simulink model "bistaticAnalysisQuickReference"  (R2026a)
settings: Solver=VariableStepAuto
settings Model: Creator=pwilliam  LastModifiedBy=pwilliam

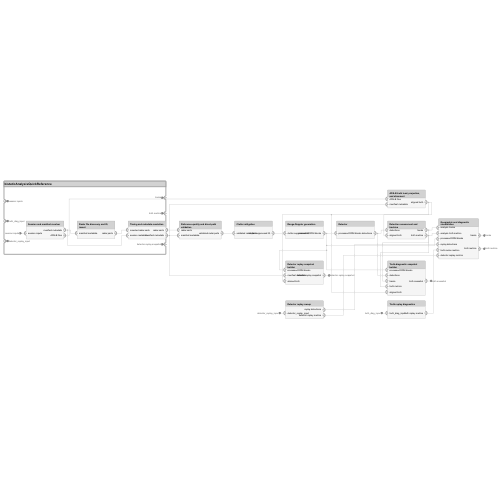
[thumbnail: Simulink's stored preview of the top-level diagram]
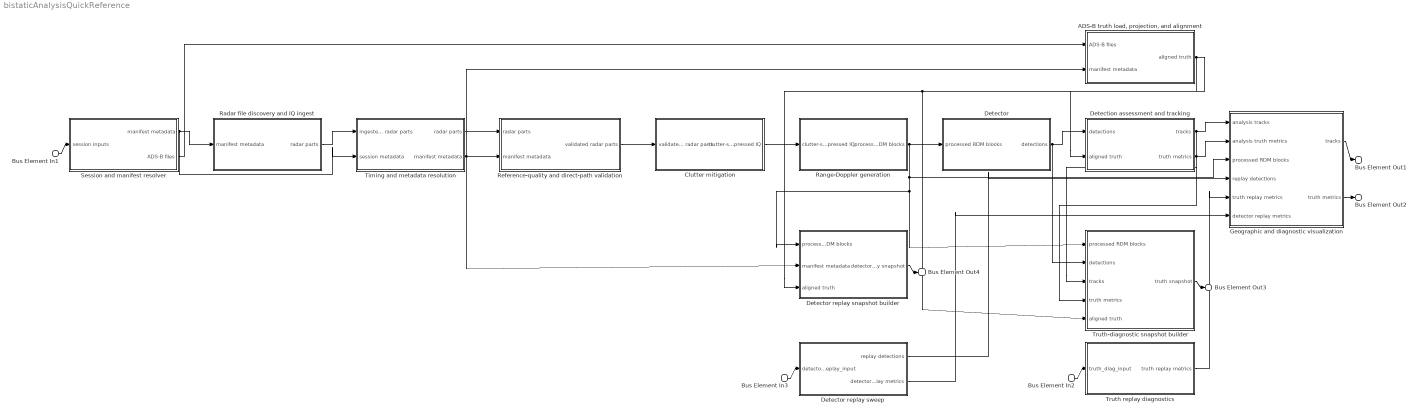
== system bistaticAnalysisQuickReference ==
  Bus Element In1 : Inport  PortName=session inputs
  Bus Element In2 : Inport  Port=2  PortName=truth_diag_input
  Bus Element In3 : Inport  Port=3  PortName=detector_replay_input
  "ADS-B truth load, projection, and alignment" : Subsystem
      settings: PortSchema="{\"entries\":[{\"content\":{\"headerSize\":26,\"margin\":15,\"minimumSpacing\":25,\"sides\":[{\"content\":{\"connectorIds\":[\"In1\",\"In2\"]},\"type\":\"ConnectorPlacement.EquallySpacedRectSide\",\"uuid\":\"3fc813c3-d4dd-4094-b53a-4fa94c312c6a\"},{\"content\":{\"connectorIds\":[\"Out1\"],\"side\":\"RIGHT\"},\"type\":\"ConnectorPlacement.EquallySpacedRectSide\",\"uuid\":\"6bc4ac0e-2abb-48a0-b5e3-8afa0902e8f2\"},{\"content\":{\"side\":\"TOP\"},\"type\":\"ConnectorPlacement.EquallySpacedRectSide\",\"uuid\":\"d3a5002a-6eae-4b58-9e29-e6d89f5a268f\"}]},\"type\":\"ConnectorPlacement.EquallySpacedConnector\",\"uuid\":\"d94812cc-5c4d-4681-a263-d12d583188a9\"}],\"packageUris\":[\"http://schema.mathworks.com/mf0/Connector/R2020b\"],\"version\":\"1.0\"}"
  Clutter mitigation : Subsystem
      settings: PortSchema="{\"entries\":[{\"content\":{\"headerSize\":26,\"margin\":15,\"minimumSpacing\":25,\"sides\":[{\"content\":{\"connectorIds\":[\"In1\"]},\"type\":\"ConnectorPlacement.EquallySpacedRectSide\",\"uuid\":\"3fc813c3-d4dd-4094-b53a-4fa94c312c6a\"},{\"content\":{\"connectorIds\":[\"Out1\"],\"side\":\"RIGHT\"},\"type\":\"ConnectorPlacement.EquallySpacedRectSide\",\"uuid\":\"6bc4ac0e-2abb-48a0-b5e3-8afa0902e8f2\"},{\"content\":{\"side\":\"TOP\"},\"type\":\"ConnectorPlacement.EquallySpacedRectSide\",\"uuid\":\"d3a5002a-6eae-4b58-9e29-e6d89f5a268f\"}]},\"type\":\"ConnectorPlacement.EquallySpacedConnector\",\"uuid\":\"d94812cc-5c4d-4681-a263-d12d583188a9\"}],\"packageUris\":[\"http://schema.mathworks.com/mf0/Connector/R2020b\"],\"version\":\"1.0\"}"
  Detection assessment and tracking : Subsystem
      settings: PortSchema="{\"entries\":[{\"content\":{\"headerSize\":26,\"margin\":15,\"minimumSpacing\":25,\"sides\":[{\"content\":{\"connectorIds\":[\"In1\",\"In2\"]},\"type\":\"ConnectorPlacement.EquallySpacedRectSide\",\"uuid\":\"3fc813c3-d4dd-4094-b53a-4fa94c312c6a\"},{\"content\":{\"connectorIds\":[\"Out1\",\"Out2\"],\"side\":\"RIGHT\"},\"type\":\"ConnectorPlacement.EquallySpacedRectSide\",\"uuid\":\"6bc4ac0e-2abb-48a0-b5e3-8afa0902e8f2\"},{\"content\":{\"side\":\"TOP\"},\"type\":\"ConnectorPlacement.EquallySpacedRectSide\",\"uuid\":\"d3a5002a-6eae-4b58-9e29-e6d89f5a268f\"}]},\"type\":\"ConnectorPlacement.EquallySpacedConnector\",\"uuid\":\"d94812cc-5c4d-4681-a263-d12d583188a9\"}],\"packageUris\":[\"http://schema.mathworks.com/mf0/Connector/R2020b\"],\"version\":\"1.0\"}"
  Detector : Subsystem
      settings: PortSchema="{\"entries\":[{\"content\":{\"headerSize\":26,\"margin\":15,\"minimumSpacing\":25,\"sides\":[{\"content\":{\"connectorIds\":[\"In1\"]},\"type\":\"ConnectorPlacement.EquallySpacedRectSide\",\"uuid\":\"3fc813c3-d4dd-4094-b53a-4fa94c312c6a\"},{\"content\":{\"connectorIds\":[\"Out1\"],\"side\":\"RIGHT\"},\"type\":\"ConnectorPlacement.EquallySpacedRectSide\",\"uuid\":\"6bc4ac0e-2abb-48a0-b5e3-8afa0902e8f2\"},{\"content\":{\"side\":\"TOP\"},\"type\":\"ConnectorPlacement.EquallySpacedRectSide\",\"uuid\":\"d3a5002a-6eae-4b58-9e29-e6d89f5a268f\"}]},\"type\":\"ConnectorPlacement.EquallySpacedConnector\",\"uuid\":\"d94812cc-5c4d-4681-a263-d12d583188a9\"}],\"packageUris\":[\"http://schema.mathworks.com/mf0/Connector/R2020b\"],\"version\":\"1.0\"}"
  Detector replay snapshot builder : Subsystem
      settings: PortSchema="{\"entries\":[{\"content\":{\"headerSize\":26,\"margin\":15,\"minimumSpacing\":25,\"sides\":[{\"content\":{\"connectorIds\":[\"In1\",\"In2\",\"In3\"]},\"type\":\"ConnectorPlacement.EquallySpacedRectSide\",\"uuid\":\"3fc813c3-d4dd-4094-b53a-4fa94c312c6a\"},{\"content\":{\"connectorIds\":[\"Out1\"],\"side\":\"RIGHT\"},\"type\":\"ConnectorPlacement.EquallySpacedRectSide\",\"uuid\":\"6bc4ac0e-2abb-48a0-b5e3-8afa0902e8f2\"},{\"content\":{\"side\":\"TOP\"},\"type\":\"ConnectorPlacement.EquallySpacedRectSide\",\"uuid\":\"d3a5002a-6eae-4b58-9e29-e6d89f5a268f\"}]},\"type\":\"ConnectorPlacement.EquallySpacedConnector\",\"uuid\":\"d94812cc-5c4d-4681-a263-d12d583188a9\"}],\"packageUris\":[\"http://schema.mathworks.com/mf0/Connector/R2020b\"],\"version\":\"1.0\"}"
  Detector replay sweep : Subsystem
      settings: PortSchema="{\"entries\":[{\"content\":{\"headerSize\":26,\"margin\":15,\"minimumSpacing\":25,\"sides\":[{\"content\":{\"connectorIds\":[\"In1\"]},\"type\":\"ConnectorPlacement.EquallySpacedRectSide\",\"uuid\":\"3fc813c3-d4dd-4094-b53a-4fa94c312c6a\"},{\"content\":{\"connectorIds\":[\"Out1\",\"Out2\"],\"side\":\"RIGHT\"},\"type\":\"ConnectorPlacement.EquallySpacedRectSide\",\"uuid\":\"6bc4ac0e-2abb-48a0-b5e3-8afa0902e8f2\"},{\"content\":{\"side\":\"TOP\"},\"type\":\"ConnectorPlacement.EquallySpacedRectSide\",\"uuid\":\"d3a5002a-6eae-4b58-9e29-e6d89f5a268f\"}]},\"type\":\"ConnectorPlacement.EquallySpacedConnector\",\"uuid\":\"d94812cc-5c4d-4681-a263-d12d583188a9\"}],\"packageUris\":[\"http://schema.mathworks.com/mf0/Connector/R2020b\"],\"version\":\"1.0\"}"
  Geographic and diagnostic visualization : Subsystem
      settings: PortSchema="{\"entries\":[{\"content\":{\"headerSize\":26,\"margin\":15,\"minimumSpacing\":25,\"sides\":[{\"content\":{\"connectorIds\":[\"In1\",\"In2\",\"In3\",\"In4\",\"In5\",\"In6\"]},\"type\":\"ConnectorPlacement.EquallySpacedRectSide\",\"uuid\":\"3fc813c3-d4dd-4094-b53a-4fa94c312c6a\"},{\"content\":{\"connectorIds\":[\"Out1\",\"Out2\"],\"side\":\"RIGHT\"},\"type\":\"ConnectorPlacement.EquallySpacedRectSide\",\"uuid\":\"6bc4ac0e-2abb-48a0-b5e3-8afa0902e8f2\"},{\"content\":{\"side\":\"TOP\"},\"type\":\"ConnectorPlacement.EquallySpacedRectSide\",\"uuid\":\"d3a5002a-6eae-4b58-9e29-e6d89f5a268f\"}]},\"type\":\"ConnectorPlacement.EquallySpacedConnector\",\"uuid\":\"d94812cc-5c4d-4681-a263-d12d583188a9\"}],\"packageUris\":[\"http://schema.mathworks.com/mf0/Connector/R2020b\"],\"version\":\"1.0\"}"
  Radar file discovery and IQ ingest : Subsystem
      settings: PortSchema="{\"entries\":[{\"content\":{\"headerSize\":26,\"margin\":15,\"minimumSpacing\":25,\"sides\":[{\"content\":{\"connectorIds\":[\"In1\"]},\"type\":\"ConnectorPlacement.EquallySpacedRectSide\",\"uuid\":\"3fc813c3-d4dd-4094-b53a-4fa94c312c6a\"},{\"content\":{\"connectorIds\":[\"Out1\"],\"side\":\"RIGHT\"},\"type\":\"ConnectorPlacement.EquallySpacedRectSide\",\"uuid\":\"6bc4ac0e-2abb-48a0-b5e3-8afa0902e8f2\"},{\"content\":{\"side\":\"TOP\"},\"type\":\"ConnectorPlacement.EquallySpacedRectSide\",\"uuid\":\"d3a5002a-6eae-4b58-9e29-e6d89f5a268f\"}]},\"type\":\"ConnectorPlacement.EquallySpacedConnector\",\"uuid\":\"d94812cc-5c4d-4681-a263-d12d583188a9\"}],\"packageUris\":[\"http://schema.mathworks.com/mf0/Connector/R2020b\"],\"version\":\"1.0\"}"
  Range-Doppler generation : Subsystem
      settings: PortSchema="{\"entries\":[{\"content\":{\"headerSize\":26,\"margin\":15,\"minimumSpacing\":25,\"sides\":[{\"content\":{\"connectorIds\":[\"In1\"]},\"type\":\"ConnectorPlacement.EquallySpacedRectSide\",\"uuid\":\"3fc813c3-d4dd-4094-b53a-4fa94c312c6a\"},{\"content\":{\"connectorIds\":[\"Out1\"],\"side\":\"RIGHT\"},\"type\":\"ConnectorPlacement.EquallySpacedRectSide\",\"uuid\":\"6bc4ac0e-2abb-48a0-b5e3-8afa0902e8f2\"},{\"content\":{\"side\":\"TOP\"},\"type\":\"ConnectorPlacement.EquallySpacedRectSide\",\"uuid\":\"d3a5002a-6eae-4b58-9e29-e6d89f5a268f\"}]},\"type\":\"ConnectorPlacement.EquallySpacedConnector\",\"uuid\":\"d94812cc-5c4d-4681-a263-d12d583188a9\"}],\"packageUris\":[\"http://schema.mathworks.com/mf0/Connector/R2020b\"],\"version\":\"1.0\"}"
  Reference-quality and direct-path validation : Subsystem
      settings: PortSchema="{\"entries\":[{\"content\":{\"headerSize\":26,\"margin\":15,\"minimumSpacing\":25,\"sides\":[{\"content\":{\"connectorIds\":[\"In1\",\"In2\"]},\"type\":\"ConnectorPlacement.EquallySpacedRectSide\",\"uuid\":\"3fc813c3-d4dd-4094-b53a-4fa94c312c6a\"},{\"content\":{\"connectorIds\":[\"Out1\"],\"side\":\"RIGHT\"},\"type\":\"ConnectorPlacement.EquallySpacedRectSide\",\"uuid\":\"6bc4ac0e-2abb-48a0-b5e3-8afa0902e8f2\"},{\"content\":{\"side\":\"TOP\"},\"type\":\"ConnectorPlacement.EquallySpacedRectSide\",\"uuid\":\"d3a5002a-6eae-4b58-9e29-e6d89f5a268f\"}]},\"type\":\"ConnectorPlacement.EquallySpacedConnector\",\"uuid\":\"d94812cc-5c4d-4681-a263-d12d583188a9\"}],\"packageUris\":[\"http://schema.mathworks.com/mf0/Connector/R2020b\"],\"version\":\"1.0\"}"
  Session and manifest resolver : Subsystem
      settings: PortSchema="{\"entries\":[{\"content\":{\"headerSize\":26,\"margin\":15,\"minimumSpacing\":25,\"sides\":[{\"content\":{\"connectorIds\":[\"In1\"]},\"type\":\"ConnectorPlacement.EquallySpacedRectSide\",\"uuid\":\"3fc813c3-d4dd-4094-b53a-4fa94c312c6a\"},{\"content\":{\"connectorIds\":[\"Out1\",\"Out2\"],\"side\":\"RIGHT\"},\"type\":\"ConnectorPlacement.EquallySpacedRectSide\",\"uuid\":\"6bc4ac0e-2abb-48a0-b5e3-8afa0902e8f2\"},{\"content\":{\"side\":\"TOP\"},\"type\":\"ConnectorPlacement.EquallySpacedRectSide\",\"uuid\":\"d3a5002a-6eae-4b58-9e29-e6d89f5a268f\"}]},\"type\":\"ConnectorPlacement.EquallySpacedConnector\",\"uuid\":\"d94812cc-5c4d-4681-a263-d12d583188a9\"}],\"packageUris\":[\"http://schema.mathworks.com/mf0/Connector/R2020b\"],\"version\":\"1.0\"}"
  Timing and metadata resolution : Subsystem
      settings: PortSchema="{\"entries\":[{\"content\":{\"headerSize\":26,\"margin\":15,\"minimumSpacing\":25,\"sides\":[{\"content\":{\"connectorIds\":[\"In1\",\"In2\"]},\"type\":\"ConnectorPlacement.EquallySpacedRectSide\",\"uuid\":\"3fc813c3-d4dd-4094-b53a-4fa94c312c6a\"},{\"content\":{\"connectorIds\":[\"Out1\",\"Out2\"],\"side\":\"RIGHT\"},\"type\":\"ConnectorPlacement.EquallySpacedRectSide\",\"uuid\":\"6bc4ac0e-2abb-48a0-b5e3-8afa0902e8f2\"},{\"content\":{\"side\":\"TOP\"},\"type\":\"ConnectorPlacement.EquallySpacedRectSide\",\"uuid\":\"d3a5002a-6eae-4b58-9e29-e6d89f5a268f\"}]},\"type\":\"ConnectorPlacement.EquallySpacedConnector\",\"uuid\":\"d94812cc-5c4d-4681-a263-d12d583188a9\"}],\"packageUris\":[\"http://schema.mathworks.com/mf0/Connector/R2020b\"],\"version\":\"1.0\"}"
  Truth replay diagnostics : Subsystem
      settings: PortSchema="{\"entries\":[{\"content\":{\"headerSize\":26,\"margin\":15,\"minimumSpacing\":25,\"sides\":[{\"content\":{\"connectorIds\":[\"In1\"]},\"type\":\"ConnectorPlacement.EquallySpacedRectSide\",\"uuid\":\"3fc813c3-d4dd-4094-b53a-4fa94c312c6a\"},{\"content\":{\"connectorIds\":[\"Out1\"],\"side\":\"RIGHT\"},\"type\":\"ConnectorPlacement.EquallySpacedRectSide\",\"uuid\":\"6bc4ac0e-2abb-48a0-b5e3-8afa0902e8f2\"},{\"content\":{\"side\":\"TOP\"},\"type\":\"ConnectorPlacement.EquallySpacedRectSide\",\"uuid\":\"d3a5002a-6eae-4b58-9e29-e6d89f5a268f\"}]},\"type\":\"ConnectorPlacement.EquallySpacedConnector\",\"uuid\":\"d94812cc-5c4d-4681-a263-d12d583188a9\"}],\"packageUris\":[\"http://schema.mathworks.com/mf0/Connector/R2020b\"],\"version\":\"1.0\"}"
  Truth-diagnostic snapshot builder : Subsystem
      settings: PortSchema="{\"entries\":[{\"content\":{\"headerSize\":26,\"margin\":15,\"minimumSpacing\":25,\"sides\":[{\"content\":{\"connectorIds\":[\"In1\",\"In2\",\"In3\",\"In4\",\"In5\"]},\"type\":\"ConnectorPlacement.EquallySpacedRectSide\",\"uuid\":\"3fc813c3-d4dd-4094-b53a-4fa94c312c6a\"},{\"content\":{\"connectorIds\":[\"Out1\"],\"side\":\"RIGHT\"},\"type\":\"ConnectorPlacement.EquallySpacedRectSide\",\"uuid\":\"6bc4ac0e-2abb-48a0-b5e3-8afa0902e8f2\"},{\"content\":{\"side\":\"TOP\"},\"type\":\"ConnectorPlacement.EquallySpacedRectSide\",\"uuid\":\"d3a5002a-6eae-4b58-9e29-e6d89f5a268f\"}]},\"type\":\"ConnectorPlacement.EquallySpacedConnector\",\"uuid\":\"d94812cc-5c4d-4681-a263-d12d583188a9\"}],\"packageUris\":[\"http://schema.mathworks.com/mf0/Connector/R2020b\"],\"version\":\"1.0\"}"
  Bus Element Out1 : Outport  PortName=tracks
  Bus Element Out2 : Outport  Port=2  PortName=truth metrics
  Bus Element Out3 : Outport  Port=3  PortName=truth snapshot
  Bus Element Out4 : Outport  Port=4  PortName=detector replay snapshot
  wires:
  Bus Element In1/1 -> Session and manifest resolver/1(session inputs)
  Session and manifest resolver/1(manifest metadata) -> Radar file discovery and IQ ingest/1(manifest metadata), Timing and metadata resolution/2(session metadata)
  Session and manifest resolver/2(ADS-B files) -> "ADS-B truth load, projection, and alignment"/1(ADS-B files)
  Radar file discovery and IQ ingest/1(radar parts) -> Timing and metadata resolution/1(ingested radar parts)
  Timing and metadata resolution/1(radar parts) -> Reference-quality and direct-path validation/1(radar parts)
  Timing and metadata resolution/2(manifest metadata) -> Reference-quality and direct-path validation/2(manifest metadata), "ADS-B truth load, projection, and alignment"/2(manifest metadata), Detector replay snapshot builder/2(manifest metadata)
  Reference-quality and direct-path validation/1(validated radar parts) -> Clutter mitigation/1(validated radar parts)
  Clutter mitigation/1(clutter-suppressed IQ) -> Range-Doppler generation/1(clutter-suppressed IQ)
  Range-Doppler generation/1(processed RDM blocks) -> Truth-diagnostic snapshot builder/1(processed RDM blocks), Detector replay snapshot builder/1(processed RDM blocks), Geographic and diagnostic visualization/3(processed RDM blocks), Detector/1(processed RDM blocks)
  Detector/1(detections) -> Detection assessment and tracking/1(detections), Truth-diagnostic snapshot builder/2(detections)
  "ADS-B truth load, projection, and alignment"/1(aligned truth) -> Detector replay snapshot builder/3(aligned truth), Truth-diagnostic snapshot builder/5(aligned truth), Detection assessment and tracking/2(aligned truth)
  Detection assessment and tracking/1(tracks) -> Geographic and diagnostic visualization/1(analysis tracks), Truth-diagnostic snapshot builder/3(tracks)
  Detection assessment and tracking/2(truth metrics) -> Geographic and diagnostic visualization/2(analysis truth metrics), Truth-diagnostic snapshot builder/4(truth metrics)
  Bus Element In2/1 -> Truth replay diagnostics/1(truth_diag_input)
  Truth replay diagnostics/1(truth replay metrics) -> Geographic and diagnostic visualization/5(truth replay metrics)
  Bus Element In3/1 -> Detector replay sweep/1(detector_replay_input)
  Detector replay sweep/1(replay detections) -> Geographic and diagnostic visualization/4(replay detections)
  Detector replay sweep/2(detector replay metrics) -> Geographic and diagnostic visualization/6(detector replay metrics)
  Geographic and diagnostic visualization/1(tracks) -> Bus Element Out1/1
  Geographic and diagnostic visualization/2(truth metrics) -> Bus Element Out2/1
  Truth-diagnostic snapshot builder/1(truth snapshot) -> Bus Element Out3/1
  Detector replay snapshot builder/1(detector replay snapshot) -> Bus Element Out4/1

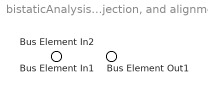
== system bistaticAnalysisQuickReference/ADS-B truth load, projection, and alignment ==
  Bus Element In1 : Inport  PortName=ADS-B files
  Bus Element In2 : Inport  Port=2  PortName=manifest metadata
  Bus Element Out1 : Outport  PortName=aligned truth

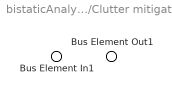
== system bistaticAnalysisQuickReference/Clutter mitigation ==
  Bus Element In1 : Inport  PortName=validated radar parts
  Bus Element Out1 : Outport  PortName=clutter-suppressed IQ

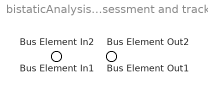
== system bistaticAnalysisQuickReference/Detection assessment and tracking ==
  Bus Element In1 : Inport  PortName=detections
  Bus Element In2 : Inport  Port=2  PortName=aligned truth
  Bus Element Out1 : Outport  PortName=tracks
  Bus Element Out2 : Outport  Port=2  PortName=truth metrics

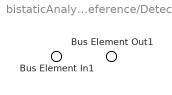
== system bistaticAnalysisQuickReference/Detector ==
  Bus Element In1 : Inport  PortName=processed RDM blocks
  Bus Element Out1 : Outport  PortName=detections

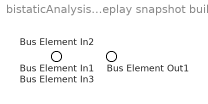
== system bistaticAnalysisQuickReference/Detector replay snapshot builder ==
  Bus Element In1 : Inport  PortName=processed RDM blocks
  Bus Element In2 : Inport  Port=2  PortName=manifest metadata
  Bus Element In3 : Inport  Port=3  PortName=aligned truth
  Bus Element Out1 : Outport  PortName=detector replay snapshot

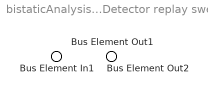
== system bistaticAnalysisQuickReference/Detector replay sweep ==
  Bus Element In1 : Inport  PortName=detector_replay_input
  Bus Element Out1 : Outport  PortName=replay detections
  Bus Element Out2 : Outport  Port=2  PortName=detector replay metrics

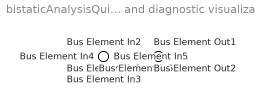
== system bistaticAnalysisQuickReference/Geographic and diagnostic visualization ==
  Bus Element In1 : Inport  PortName=analysis tracks
  Bus Element In2 : Inport  Port=2  PortName=analysis truth metrics
  Bus Element In3 : Inport  Port=3  PortName=processed RDM blocks
  Bus Element In4 : Inport  Port=4  PortName=replay detections
  Bus Element In5 : Inport  Port=5  PortName=truth replay metrics
  Bus Element In6 : Inport  Port=6  PortName=detector replay metrics
  Bus Element Out1 : Outport  PortName=tracks
  Bus Element Out2 : Outport  Port=2  PortName=truth metrics

== system bistaticAnalysisQuickReference/Radar file discovery and IQ ingest ==
  Bus Element In1 : Inport  PortName=manifest metadata
  Bus Element Out1 : Outport  PortName=radar parts

== system bistaticAnalysisQuickReference/Range-Doppler generation ==
  Bus Element In1 : Inport  PortName=clutter-suppressed IQ
  Bus Element Out1 : Outport  PortName=processed RDM blocks

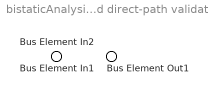
== system bistaticAnalysisQuickReference/Reference-quality and direct-path validation ==
  Bus Element In1 : Inport  PortName=radar parts
  Bus Element In2 : Inport  Port=2  PortName=manifest metadata
  Bus Element Out1 : Outport  PortName=validated radar parts

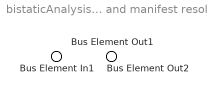
== system bistaticAnalysisQuickReference/Session and manifest resolver ==
  Bus Element In1 : Inport  PortName=session inputs
  Bus Element Out1 : Outport  PortName=manifest metadata
  Bus Element Out2 : Outport  Port=2  PortName=ADS-B files

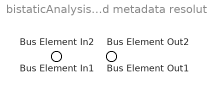
== system bistaticAnalysisQuickReference/Timing and metadata resolution ==
  Bus Element In1 : Inport  PortName=ingested radar parts
  Bus Element In2 : Inport  Port=2  PortName=session metadata
  Bus Element Out1 : Outport  PortName=radar parts
  Bus Element Out2 : Outport  Port=2  PortName=manifest metadata

== system bistaticAnalysisQuickReference/Truth replay diagnostics ==
  Bus Element In1 : Inport  PortName=truth_diag_input
  Bus Element Out1 : Outport  PortName=truth replay metrics

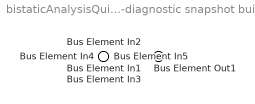
== system bistaticAnalysisQuickReference/Truth-diagnostic snapshot builder ==
  Bus Element In1 : Inport  PortName=processed RDM blocks
  Bus Element In2 : Inport  Port=2  PortName=detections
  Bus Element In3 : Inport  Port=3  PortName=tracks
  Bus Element In4 : Inport  Port=4  PortName=truth metrics
  Bus Element In5 : Inport  Port=5  PortName=aligned truth
  Bus Element Out1 : Outport  PortName=truth snapshot
